simulink model "Xl_ch16_LPF_int_v4"  (Simulink 7.5)
settings: Solver=VariableStepDiscrete  StartTime=0.0  StopTime=0.001  RelTol=1e-3
values from neighbouring files (symbols this model uses):
  a2a = zeros(nFc, length(Hd.sosMatrix(:,5)))    [iirButter_SOS_init_v2.m]    (also in iirButter_SOS_init_v2_8pole.m)
  a3a = zeros(nFc, length(Hd.sosMatrix(:,6)))    [iirButter_SOS_init_v2.m]    (also in iirButter_SOS_init_v2_8pole.m)
  dt = 1/Fsim    (= 2.56e-06)    [iirButter_SOS_init_v2.m]    (also in iirButter_SOS_init_v2_8pole.m)
  Fc_min = 10    [iirButter_SOS_init_v2.m]    (also in iirButter_SOS_init_v2_8pole.m)
  ga = zeros(nFc, length(Hd.ScaleValues))    [iirButter_SOS_init_v2.m]    (also in iirButter_SOS_init_v2_8pole.m = zeros(nFc, length(Hd.ScaleValues(1:end-1))))
  rFc = (Fc_max/Fc_min)^(1/(nFc - 1))    (= 1.70532863139)    [iirButter_SOS_init_v2.m]    (also in iirButter_SOS_init_v2_8pole.m)
  Sra = 2^34|.02  |.027 |.027 |<.038| 1e-6|<2e-6|<2e-6|<2e-6|<2e-6| 8e-6|    [iirButter_SOS_init_v2.m]    (also in iirButter_SOS_init_v2_8pole.m)
  Srm = 2^34|     |     |     |     |     |     |     |     |     |  to |    [iirButter_SOS_init_v2.m]    (also in iirButter_SOS_init_v2_8pole.m)
libraries: xbsIndex_r4 x296, dspsrcs4 x16, simulink x9
(part 2 of 2)

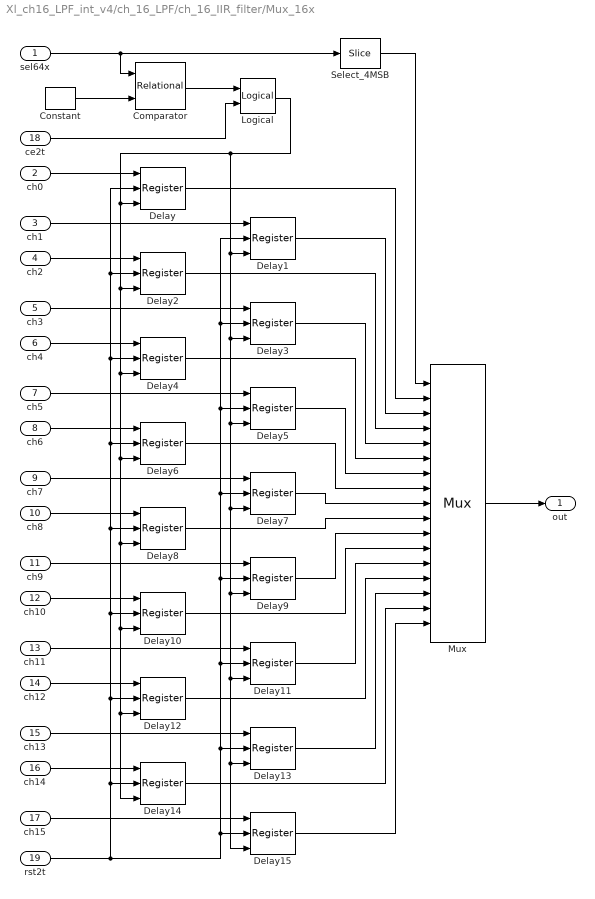
== system Xl_ch16_LPF_int_v4/ch_16_LPF/ch_16_IIR_filter/Mux_16x ==
  sel64x : Inport  OutDataType=fixdt(1, 16)  OutScaling=2^0
  ch0 : Inport  Port=2  OutDataType=fixdt(1, 16)  OutScaling=2^0
  ch1 : Inport  Port=3  OutDataType=fixdt(1, 16)  OutScaling=2^0
  ch2 : Inport  Port=4  OutDataType=fixdt(1, 16)  OutScaling=2^0
  ch3 : Inport  Port=5  OutDataType=fixdt(1, 16)  OutScaling=2^0
  ch4 : Inport  Port=6  OutDataType=fixdt(1, 16)  OutScaling=2^0
  ch5 : Inport  Port=7  OutDataType=fixdt(1, 16)  OutScaling=2^0
  ch6 : Inport  Port=8  OutDataType=fixdt(1, 16)  OutScaling=2^0
  ch7 : Inport  Port=9  OutDataType=fixdt(1, 16)  OutScaling=2^0
  ch8 : Inport  Port=10  OutDataType=fixdt(1, 16)  OutScaling=2^0
  ch9 : Inport  Port=11  OutDataType=fixdt(1, 16)  OutScaling=2^0
  ch10 : Inport  Port=12  OutDataType=fixdt(1, 16)  OutScaling=2^0
  ch11 : Inport  Port=13  OutDataType=fixdt(1, 16)  OutScaling=2^0
  ch12 : Inport  Port=14  OutDataType=fixdt(1, 16)  OutScaling=2^0
  ch13 : Inport  Port=15  OutDataType=fixdt(1, 16)  OutScaling=2^0
  ch14 : Inport  Port=16  OutDataType=fixdt(1, 16)  OutScaling=2^0
  ch15 : Inport  Port=17  OutDataType=fixdt(1, 16)  OutScaling=2^0
  ce2t : Inport  Port=18  OutDataType=fixdt(1, 16)  OutScaling=2^0
  rst2t : Inport  Port=19  OutDataType=fixdt(1, 16)  OutScaling=2^0
  Comparator : xbsIndex_r4/Relational  mode=a=b  en=off  latency=0  dbl_ovrd=off  block_type=relational
      settings: block_version=12.2
  Constant : xbsIndex_r4/Constant  arith_type=Unsigned  const=63  n_bits=6  bin_pt=0  explicit_period=off  period=1  equ=P=C  opselect=C  inp2=PCIN>>17  opr=+  inp1=P  carry=CIN  dbl_ovrd=off  block_type=constant
      settings: block_version=12.2
  Delay{,1..15} (16 alike) : xbsIndex_r4/Register  init=0  rst=on  en=on  dbl_ovrd=off  block_type=register
      settings: block_version=12.2
  Logical : xbsIndex_r4/Logical  logical_function=AND  inputs=2  en=off  latency=0  precision=Full  arith_type=Unsigned  n_bits=16  bin_pt=0  align_bp=on  dbl_ovrd=off  block_type=logical
      settings: block_version=12.2
  Mux : xbsIndex_r4/Mux  inputs=16  en=off  latency=0  precision=Full  arith_type=Unsigned  n_bits=16  bin_pt=14  quantization=Truncate  overflow=Wrap  dbl_ovrd=off  block_type=mux
      settings: block_version=12.2
  Select_4MSB : xbsIndex_r4/Slice  nbits=4  boolean_output=off  mode=Upper Bit Location + Width  bit1=0  base1=MSB of Input  bit0=0  base0=LSB of Input  dbl_ovrd=off  block_type=slice
      settings: block_version=12.2
  out : Outport  OutDataType=fixdt(1, 16)  OutScaling=2^0
  wires:
  Select_4MSB/1 -> Mux/1
  Delay14/1 -> Mux/16
  Delay13/1 -> Mux/15
  Delay12/1 -> Mux/14
  Delay11/1 -> Mux/13
  Delay10/1 -> Mux/12
  Delay9/1 -> Mux/11
  Delay1/1 -> Mux/3
  Delay2/1 -> Mux/4
  Delay3/1 -> Mux/5
  Delay4/1 -> Mux/6
  Delay5/1 -> Mux/7
  Delay6/1 -> Mux/8
  Delay7/1 -> Mux/9
  Delay8/1 -> Mux/10
  Delay/1 -> Mux/2
  Delay15/1 -> Mux/17
  rst2t/1 -> Delay14/2, Delay12/2, Delay10/2, Delay8/2, Delay6/2, Delay4/2, Delay2/2, Delay/2, Delay3/2, Delay1/2, Delay5/2, Delay7/2, Delay9/2, Delay11/2, Delay13/2, Delay15/2
  Logical/1 -> Delay/3, Delay2/3, Delay4/3, Delay6/3, Delay8/3, Delay10/3, Delay12/3, Delay14/3, Delay13/3, Delay15/3, Delay11/3, Delay9/3, Delay7/3, Delay5/3, Delay3/3, Delay1/3
  ce2t/1 -> Logical/2
  Comparator/1 -> Logical/1
  ch15/1 -> Delay15/1
  ch14/1 -> Delay14/1
  ch13/1 -> Delay13/1
  ch12/1 -> Delay12/1
  ch11/1 -> Delay11/1
  ch10/1 -> Delay10/1
  ch9/1 -> Delay9/1
  ch8/1 -> Delay8/1
  ch7/1 -> Delay7/1
  ch6/1 -> Delay6/1
  ch5/1 -> Delay5/1
  ch4/1 -> Delay4/1
  sel64x/1 -> Comparator/1, Select_4MSB/1
  ch3/1 -> Delay3/1
  ch2/1 -> Delay2/1
  ch1/1 -> Delay1/1
  ch0/1 -> Delay/1
  Mux/1 -> out/1
  Constant/1 -> Comparator/2

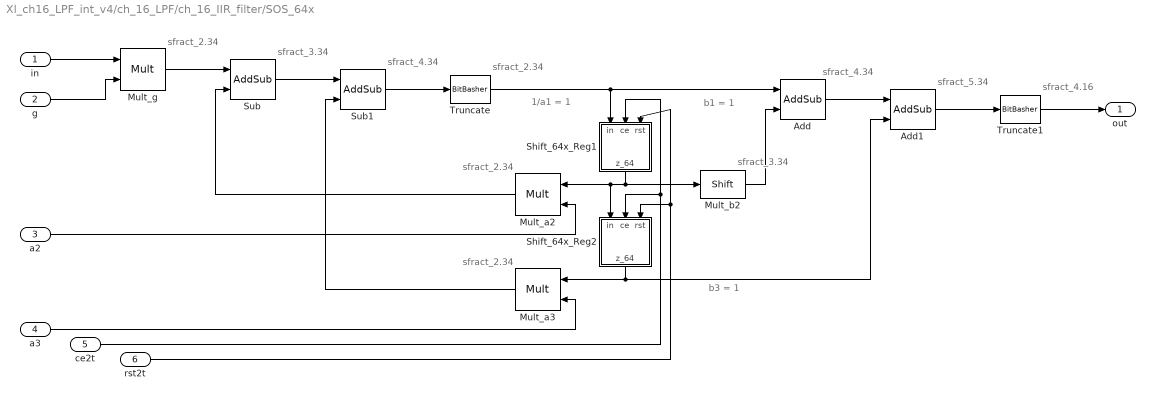
== system Xl_ch16_LPF_int_v4/ch_16_LPF/ch_16_IIR_filter/SOS_64x ==
  note: b1 = 1
  note: b3 = 1
  note: 1/a1 = 1
  note: sfract_3.34
  note: sfract_4.34
  note: sfract_2.34
  note: sfract_3.34
  note: sfract_4.34
  note: sfract_2.34
  note: sfract_2.34
  note: sfract_2.34
  note: sfract_5.34
  note: sfract_4.16
  in : Inport
  g : Inport  Port=2
  a2 : Inport  Port=3
  a3 : Inport  Port=4
  ce2t : Inport  Port=5
  rst2t : Inport  Port=6
  Add : xbsIndex_r4/AddSub  mode=Addition  use_carryin=off  use_carryout=off  en=off  latency=0  precision=Full  arith_type=Unsigned  n_bits=16  bin_pt=14  quantization=Truncate  overflow=Wrap  dbl_ovrd=off  use_behavioral_HDL=off  hw_selection=Fabric  pipelined=off  block_type=addsub
      settings: block_version=12.2
  Add1 : xbsIndex_r4/AddSub  mode=Addition  use_carryin=off  use_carryout=off  en=off  latency=0  precision=Full  arith_type=Unsigned  n_bits=16  bin_pt=14  quantization=Truncate  overflow=Wrap  dbl_ovrd=off  use_behavioral_HDL=off  hw_selection=Fabric  pipelined=off  block_type=addsub
      settings: block_version=12.2
  Mult_a2 : xbsIndex_r4/Mult  precision=User Defined  arith_type="Signed  (2's comp)"  n_bits=36  bin_pt=34  quantization=Truncate  overflow=Wrap  en=off  latency=0  dbl_ovrd=off  use_behavioral_HDL=off  opt=Speed  use_embedded=on  optimum_pipeline=off  pipeline=on  use_rpm=on  placement_style=Triangular  block_type=mult
      settings: block_version=12.2
  Mult_a3 : xbsIndex_r4/Mult  precision=User Defined  arith_type="Signed  (2's comp)"  n_bits=36  bin_pt=34  quantization=Truncate  overflow=Wrap  en=off  latency=0  dbl_ovrd=off  use_behavioral_HDL=off  opt=Speed  use_embedded=on  optimum_pipeline=off  pipeline=on  use_rpm=on  placement_style=Triangular  block_type=mult
      settings: block_version=12.2
  Mult_b2 : xbsIndex_r4/Shift  shift_dir=Left  shift_bits=1  en=off  latency=0  precision=User Defined  arith_type="Signed  (2's comp)"  n_bits=37  bin_pt=34  quantization=Truncate  overflow=Wrap  dbl_ovrd=off  block_type=shift
      settings: block_version=12.2
  Mult_g : xbsIndex_r4/Mult  precision=User Defined  arith_type="Signed  (2's comp)"  n_bits=36  bin_pt=34  quantization=Truncate  overflow=Wrap  en=off  latency=0  dbl_ovrd=off  use_behavioral_HDL=off  opt=Speed  use_embedded=on  optimum_pipeline=off  pipeline=on  use_rpm=on  placement_style=Triangular  block_type=mult
      settings: block_version=12.2
  Shift_64x_Reg1 : Subsystem
  Shift_64x_Reg2 : Subsystem
  Sub : xbsIndex_r4/AddSub  mode=Subtraction  use_carryin=off  use_carryout=off  en=off  latency=0  precision=Full  arith_type=Unsigned  n_bits=16  bin_pt=14  quantization=Truncate  overflow=Wrap  dbl_ovrd=off  use_behavioral_HDL=off  hw_selection=Fabric  pipelined=off  block_type=addsub
      settings: block_version=12.2
  Sub1 : xbsIndex_r4/AddSub  mode=Subtraction  use_carryin=off  use_carryout=off  en=off  latency=0  precision=Full  arith_type=Unsigned  n_bits=16  bin_pt=14  quantization=Truncate  overflow=Wrap  dbl_ovrd=off  use_behavioral_HDL=off  hw_selection=Fabric  pipelined=off  block_type=addsub
      settings: block_version=12.2
  Truncate : xbsIndex_r4/BitBasher  bitexpr=|  display_expr=off  sr_1=1  arith_type1="Signed  (2's comp)"  bin_pt1=34  sr_2=2  arith_type2=Unsigned  bin_pt2=0  sr_3=3  arith_type3=Unsigned  bin_pt3=0  sr_4=4  arith_type4=Unsigned  bin_pt4=0  dbl_ovrd=off  block_type=bitbasher
      | <!DOCTYPE HTML PUBLIC "-//W3C//DTD HTML 4.0//EN" "http://www.w3.org/TR/REC-html40/strict.dtd">
      | <html><head><meta name="qrichtext" content="1" /><style type="text/css">
      | p, li { white-space: pre-wrap; }
      | </style></head><body style=" font-family:'MS Shell Dlg 2'; font-size:8.25pt; font-weight:400; font-style:normal;">
      | <p style=" margin-top:12px; margin-bottom:12px; margin-left:0px; margin-right:0px; -qt-block-indent:0; text-indent:0px; font-family:'MS Shell Dlg'; font-size:8pt;">a={b[35:0]}</p></body></html>
      settings: block_version=12.2
  Truncate1 : xbsIndex_r4/BitBasher  bitexpr=|  display_expr=off  sr_1=1  arith_type1="Signed  (2's comp)"  bin_pt1=16  sr_2=2  arith_type2=Unsigned  bin_pt2=0  sr_3=3  arith_type3=Unsigned  bin_pt3=0  sr_4=4  arith_type4=Unsigned  bin_pt4=0  dbl_ovrd=off  block_type=bitbasher
      | <!DOCTYPE HTML PUBLIC "-//W3C//DTD HTML 4.0//EN" "http://www.w3.org/TR/REC-html40/strict.dtd">
      | <html><head><meta name="qrichtext" content="1" /><style type="text/css">
      | p, li { white-space: pre-wrap; }
      | </style></head><body style=" font-family:'MS Shell Dlg 2'; font-size:8.25pt; font-weight:400; font-style:normal;">
      | <p style=" margin-top:12px; margin-bottom:12px; margin-left:0px; margin-right:0px; -qt-block-indent:0; text-indent:0px; font-family:'MS Shell Dlg'; font-size:8pt;">a={b[37:18]}</p></body></html>
      settings: block_version=12.2
  out : Outport
  wires:
  a3/1 -> Mult_a3/2
  a2/1 -> Mult_a2/2
  g/1 -> Mult_g/2
  Shift_64x_Reg1/1(z_64) -> Mult_a2/1, Shift_64x_Reg2/1(in), Mult_b2/1
  Mult_b2/1 -> Add/2
  Shift_64x_Reg2/1(z_64) -> Mult_a3/1, Add1/2
  Sub1/1 -> Truncate/1
  Mult_a2/1 -> Sub/2
  Mult_a3/1 -> Sub1/2
  Mult_g/1 -> Sub/1
  in/1 -> Mult_g/1
  Add1/1 -> Truncate1/1
  Truncate/1 -> Add/1, Shift_64x_Reg1/1(in)
  Truncate1/1 -> out/1
  Add/1 -> Add1/1
  Sub/1 -> Sub1/1
  ce2t/1 -> Shift_64x_Reg1/2(ce), Shift_64x_Reg2/2(ce)
  rst2t/1 -> Shift_64x_Reg1/3(rst), Shift_64x_Reg2/3(rst)

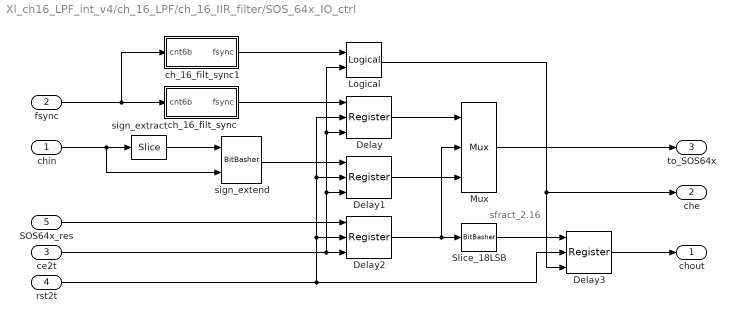
== system Xl_ch16_LPF_int_v4/ch_16_LPF/ch_16_IIR_filter/SOS_64x_IO_ctrl ==
  note: sfract_2.16
  chin : Inport  OutDataType=fixdt(1, 16)  OutScaling=2^0
  fsync : Inport  Port=2  OutDataType=fixdt(1, 16)  OutScaling=2^0
  ce2t : Inport  Port=3  OutDataType=fixdt(1, 16)  OutScaling=2^0
  rst2t : Inport  Port=4  OutDataType=fixdt(1, 16)  OutScaling=2^0
  SOS64x_res : Inport  Port=5  OutDataType=fixdt(1, 16)  OutScaling=2^0
  Delay{,1..3} (4 alike) : xbsIndex_r4/Register  init=0  rst=on  en=on  dbl_ovrd=off  block_type=register
      settings: block_version=12.2
  Logical : xbsIndex_r4/Logical  logical_function=AND  inputs=2  en=off  latency=0  precision=Full  arith_type=Unsigned  n_bits=16  bin_pt=0  align_bp=on  dbl_ovrd=off  block_type=logical
      settings: block_version=12.2
  Mux : xbsIndex_r4/Mux  inputs=2  en=off  latency=0  precision=Full  arith_type=Unsigned  n_bits=16  bin_pt=14  quantization=Truncate  overflow=Wrap  dbl_ovrd=off  block_type=mux
      settings: block_version=12.2
  Slice_18LSB : xbsIndex_r4/BitBasher  bitexpr=|  display_expr=off  sr_1=1  arith_type1="Signed  (2's comp)"  bin_pt1=16  sr_2=2  arith_type2=Unsigned  bin_pt2=0  sr_3=3  arith_type3=Unsigned  bin_pt3=0  sr_4=4  arith_type4=Unsigned  bin_pt4=0  dbl_ovrd=off  block_type=bitbasher
      | <!DOCTYPE HTML PUBLIC "-//W3C//DTD HTML 4.0//EN" "http://www.w3.org/TR/REC-html40/strict.dtd">
      | <html><head><meta name="qrichtext" content="1" /><style type="text/css">
      | p, li { white-space: pre-wrap; }
      | </style></head><body style=" font-family:'MS Shell Dlg 2'; font-size:8.25pt; font-weight:400; font-style:normal;">
      | <p style=" margin-top:12px; margin-bottom:12px; margin-left:0px; margin-right:0px; -qt-block-indent:0; text-indent:0px; font-family:'MS Shell Dlg'; font-size:8pt;">a={b[17:0]}</p></body></html>
      settings: block_version=12.2
  ch_16_filt_sync : Subsystem
  ch_16_filt_sync1 : Subsystem
  sign_extend : xbsIndex_r4/BitBasher  bitexpr=|  display_expr=off  sr_1=1  arith_type1="Signed  (2's comp)"  bin_pt1=16  sr_2=2  arith_type2=Unsigned  bin_pt2=0  sr_3=3  arith_type3=Unsigned  bin_pt3=0  sr_4=4  arith_type4=Unsigned  bin_pt4=0  dbl_ovrd=off  block_type=bitbasher
      | <!DOCTYPE HTML PUBLIC "-//W3C//DTD HTML 4.0//EN" "http://www.w3.org/TR/REC-html40/strict.dtd">
      | <html><head><meta name="qrichtext" content="1" /><style type="text/css">
      | p, li { white-space: pre-wrap; }
      | </style></head><body style=" font-family:'MS Shell Dlg 2'; font-size:8.25pt; font-weight:400; font-style:normal;">
      | <p style=" margin-top:12px; margin-bottom:12px; margin-left:0px; margin-right:0px; -qt-block-indent:0; text-indent:0px; font-family:'MS Shell Dlg'; font-size:8pt;">a={2{b},c}</p></body></html>
      settings: block_version=12.2
  sign_extract : xbsIndex_r4/Slice  nbits=1  boolean_output=on  mode=Upper Bit Location + Width  bit1=0  base1=MSB of Input  bit0=0  base0=LSB of Input  dbl_ovrd=off  block_type=slice
      settings: block_version=12.2
  chout : Outport  OutDataType=fixdt(1, 16)  OutScaling=2^0
  che : Outport  Port=2  OutDataType=fixdt(1, 16)  OutScaling=2^0
  to_SOS64x : Outport  Port=3  OutDataType=fixdt(1, 16)  OutScaling=2^0
  wires:
  fsync/1 -> ch_16_filt_sync/1(cnt6b), ch_16_filt_sync1/1(cnt6b)
  Delay/1 -> Mux/1
  Delay1/1 -> Mux/3
  chin/1 -> sign_extract/1, sign_extend/2
  Delay2/1 -> Mux/2, Slice_18LSB/1
  SOS64x_res/1 -> Delay2/1
  Mux/1 -> to_SOS64x/1
  Logical/1 -> Delay3/3, che/1
  ce2t/1 -> Delay2/3, Delay/3, Logical/2, Delay1/3
  rst2t/1 -> Delay/2, Delay1/2, Delay2/2, Delay3/2
  sign_extend/1 -> Delay1/1
  sign_extract/1 -> sign_extend/1
  Slice_18LSB/1 -> Delay3/1
  ch_16_filt_sync/1(fsync) -> Delay/1
  ch_16_filt_sync1/1(fsync) -> Logical/1
  Delay3/1 -> chout/1

== system Xl_ch16_LPF_int_v4/ch_16_LPF/ch_16_IIR_filter/Subsystem ==
  In1 : Inport
  Time Division Demultiplexer : xbsIndex_r4/Time Division Demultiplexer  frame_pattern=[1 0]  impl_style=Multiple Channel  vin=off  dbl_ovrd=off  explicit_period=off  period=1  block_type=tdd
      settings: infoedit=Samples presented at the input are selected and down-sampled according to the frame sampling pattern specified. The sampled input is presented either as a single or multiple channel at the output.  block_version=12.2
  Time Division Demultiplexer1 : xbsIndex_r4/Time Division Demultiplexer  frame_pattern=[0 0 0 1 1 0 0 0 zeros(1,24)]  impl_style=Multiple Channel  vin=off  dbl_ovrd=off  explicit_period=off  period=1  block_type=tdd
      settings: infoedit=Samples presented at the input are selected and down-sampled according to the frame sampling pattern specified. The sampled input is presented either as a single or multiple channel at the output.  block_version=12.2
  Time Division Demultiplexer2 : xbsIndex_r4/Time Division Demultiplexer  frame_pattern=[1 1]  impl_style=Multiple Channel  vin=off  dbl_ovrd=off  explicit_period=off  period=1  block_type=tdd
      settings: infoedit=Samples presented at the input are selected and down-sampled according to the frame sampling pattern specified. The sampled input is presented either as a single or multiple channel at the output.  block_version=12.2
  Time Division Demultiplexer3 : xbsIndex_r4/Time Division Demultiplexer  frame_pattern=[0 0 0 1 1 0 0 0 zeros(1,24)]  impl_style=Multiple Channel  vin=off  dbl_ovrd=off  explicit_period=off  period=1  block_type=tdd
      settings: infoedit=Samples presented at the input are selected and down-sampled according to the frame sampling pattern specified. The sampled input is presented either as a single or multiple channel at the output.  block_version=12.2
  Out1 : Outport
  Out2 : Outport  Port=2
  Out3 : Outport  Port=3
  Out4 : Outport  Port=4
  wires:
  Time Division Demultiplexer/1 -> Time Division Demultiplexer2/1
  Time Division Demultiplexer2/1 -> Time Division Demultiplexer1/1
  Time Division Demultiplexer2/2 -> Time Division Demultiplexer3/1
  Time Division Demultiplexer1/1 -> Out1/1
  In1/1 -> Time Division Demultiplexer/1
  Time Division Demultiplexer1/2 -> Out2/1
  Time Division Demultiplexer3/1 -> Out3/1
  Time Division Demultiplexer3/2 -> Out4/1

== system Xl_ch16_LPF_int_v4/ch_16_LPF/ch_16_IIR_filter/Subsystem1 ==
  In1 : Inport
  Time Division Demultiplexer : xbsIndex_r4/Time Division Demultiplexer  frame_pattern=[1 0]  impl_style=Multiple Channel  vin=off  dbl_ovrd=off  explicit_period=off  period=1  block_type=tdd
      settings: infoedit=Samples presented at the input are selected and down-sampled according to the frame sampling pattern specified. The sampled input is presented either as a single or multiple channel at the output.  block_version=12.2
  Time Division Demultiplexer1 : xbsIndex_r4/Time Division Demultiplexer  frame_pattern=[0 0 0 1 1 0 0 0 zeros(1,24)]  impl_style=Multiple Channel  vin=off  dbl_ovrd=off  explicit_period=off  period=1  block_type=tdd
      settings: infoedit=Samples presented at the input are selected and down-sampled according to the frame sampling pattern specified. The sampled input is presented either as a single or multiple channel at the output.  block_version=12.2
  Time Division Demultiplexer2 : xbsIndex_r4/Time Division Demultiplexer  frame_pattern=[1 1]  impl_style=Multiple Channel  vin=off  dbl_ovrd=off  explicit_period=off  period=1  block_type=tdd
      settings: infoedit=Samples presented at the input are selected and down-sampled according to the frame sampling pattern specified. The sampled input is presented either as a single or multiple channel at the output.  block_version=12.2
  Time Division Demultiplexer3 : xbsIndex_r4/Time Division Demultiplexer  frame_pattern=[0 0 0 1 1 0 0 0 zeros(1,24)]  impl_style=Multiple Channel  vin=off  dbl_ovrd=off  explicit_period=off  period=1  block_type=tdd
      settings: infoedit=Samples presented at the input are selected and down-sampled according to the frame sampling pattern specified. The sampled input is presented either as a single or multiple channel at the output.  block_version=12.2
  Out1 : Outport
  Out2 : Outport  Port=2
  Out3 : Outport  Port=3
  Out4 : Outport  Port=4
  wires:
  Time Division Demultiplexer/1 -> Time Division Demultiplexer2/1
  Time Division Demultiplexer2/1 -> Time Division Demultiplexer1/1
  Time Division Demultiplexer2/2 -> Time Division Demultiplexer3/1
  Time Division Demultiplexer1/1 -> Out1/1
  In1/1 -> Time Division Demultiplexer/1
  Time Division Demultiplexer1/2 -> Out2/1
  Time Division Demultiplexer3/1 -> Out3/1
  Time Division Demultiplexer3/2 -> Out4/1

== system Xl_ch16_LPF_int_v4/ch_16_LPF/ch_16_IIR_filter/Subsystem2 ==
  In1 : Inport
  Time Division Demultiplexer : xbsIndex_r4/Time Division Demultiplexer  frame_pattern=[1 0]  impl_style=Multiple Channel  vin=off  dbl_ovrd=off  explicit_period=off  period=1  block_type=tdd
      settings: infoedit=Samples presented at the input are selected and down-sampled according to the frame sampling pattern specified. The sampled input is presented either as a single or multiple channel at the output.  block_version=12.2
  Time Division Demultiplexer1 : xbsIndex_r4/Time Division Demultiplexer  frame_pattern=[0 0 0 1 1 1 0 0 zeros(1,24)]  impl_style=Multiple Channel  vin=off  dbl_ovrd=off  explicit_period=off  period=1  block_type=tdd
      settings: infoedit=Samples presented at the input are selected and down-sampled according to the frame sampling pattern specified. The sampled input is presented either as a single or multiple channel at the output.  block_version=12.2
  Time Division Demultiplexer2 : xbsIndex_r4/Time Division Demultiplexer  frame_pattern=[1 1]  impl_style=Multiple Channel  vin=off  dbl_ovrd=off  explicit_period=off  period=1  block_type=tdd
      settings: infoedit=Samples presented at the input are selected and down-sampled according to the frame sampling pattern specified. The sampled input is presented either as a single or multiple channel at the output.  block_version=12.2
  Time Division Demultiplexer3 : xbsIndex_r4/Time Division Demultiplexer  frame_pattern=[0 0 0 1 1 1 0 0 zeros(1,24)]  impl_style=Multiple Channel  vin=off  dbl_ovrd=off  explicit_period=off  period=1  block_type=tdd
      settings: infoedit=Samples presented at the input are selected and down-sampled according to the frame sampling pattern specified. The sampled input is presented either as a single or multiple channel at the output.  block_version=12.2
  Out1 : Outport
  Out2 : Outport  Port=2
  Out3 : Outport  Port=3
  Out4 : Outport  Port=4
  Out5 : Outport  Port=5
  Out6 : Outport  Port=6
  wires:
  Time Division Demultiplexer/1 -> Time Division Demultiplexer2/1
  Time Division Demultiplexer2/1 -> Time Division Demultiplexer1/1
  Time Division Demultiplexer2/2 -> Time Division Demultiplexer3/1
  Time Division Demultiplexer1/1 -> Out1/1
  In1/1 -> Time Division Demultiplexer/1
  Time Division Demultiplexer1/2 -> Out2/1
  Time Division Demultiplexer3/1 -> Out3/1
  Time Division Demultiplexer3/2 -> Out4/1
  Time Division Demultiplexer1/3 -> Out5/1
  Time Division Demultiplexer3/3 -> Out6/1

== system Xl_ch16_LPF_int_v4/ch_16_LPF/ch_16_IIR_filter/ch_16_filt_sync1 ==
  cnt6b : Inport  OutDataType=fixdt(1, 16)  OutScaling=2^0
  ce2t : Inport  Port=2  OutDataType=fixdt(1, 16)  OutScaling=2^0
  AeqB : xbsIndex_r4/Relational  mode=a=b  en=off  latency=0  dbl_ovrd=off  block_type=relational
      settings: block_version=12.2
  Constant : xbsIndex_r4/Constant  arith_type=Unsigned  const=2  n_bits=2  bin_pt=0  explicit_period=off  period=1  equ=P=C  opselect=C  inp2=PCIN>>17  opr=+  inp1=P  carry=CIN  dbl_ovrd=off  block_type=constant
      settings: block_version=12.2
  Logical : xbsIndex_r4/Logical  logical_function=AND  inputs=2  en=off  latency=0  precision=Full  arith_type=Unsigned  n_bits=16  bin_pt=0  align_bp=on  dbl_ovrd=off  block_type=logical
      settings: block_version=12.2
  Slice_2LSB : xbsIndex_r4/Slice  nbits=2  boolean_output=off  mode=Lower Bit Location + Width  bit1=0  base1=MSB of Input  bit0=0  base0=LSB of Input  dbl_ovrd=off  block_type=slice
      settings: block_version=12.2
  fsync : Outport  OutDataType=fixdt(1, 16)  OutScaling=2^0
  che : Outport  Port=2  OutDataType=fixdt(1, 16)  OutScaling=2^0
  wires:
  cnt6b/1 -> Slice_2LSB/1
  Slice_2LSB/1 -> AeqB/1
  AeqB/1 -> fsync/1, Logical/1
  Constant/1 -> AeqB/2
  ce2t/1 -> Logical/2
  Logical/1 -> che/1

== system Xl_ch16_LPF_int_v4/ch_16_LPF/ch_16_IIR_filter/Demux_16x/Subsystem1 ==
  In1 : Inport
  Time Division Demultiplexer : xbsIndex_r4/Time Division Demultiplexer  frame_pattern=[1 0]  impl_style=Multiple Channel  vin=off  dbl_ovrd=off  explicit_period=off  period=1  block_type=tdd
      settings: infoedit=Samples presented at the input are selected and down-sampled according to the frame sampling pattern specified. The sampled input is presented either as a single or multiple channel at the output.  block_version=12.2
  Time Division Demultiplexer1 : xbsIndex_r4/Time Division Demultiplexer  frame_pattern=[0 0 0 1 1 1 0 0 zeros(1,24)]  impl_style=Multiple Channel  vin=off  dbl_ovrd=off  explicit_period=off  period=1  block_type=tdd
      settings: infoedit=Samples presented at the input are selected and down-sampled according to the frame sampling pattern specified. The sampled input is presented either as a single or multiple channel at the output.  block_version=12.2
  Time Division Demultiplexer2 : xbsIndex_r4/Time Division Demultiplexer  frame_pattern=[1 1]  impl_style=Multiple Channel  vin=off  dbl_ovrd=off  explicit_period=off  period=1  block_type=tdd
      settings: infoedit=Samples presented at the input are selected and down-sampled according to the frame sampling pattern specified. The sampled input is presented either as a single or multiple channel at the output.  block_version=12.2
  Time Division Demultiplexer3 : xbsIndex_r4/Time Division Demultiplexer  frame_pattern=[0 0 0 1 1 1 0 0 zeros(1,24)]  impl_style=Multiple Channel  vin=off  dbl_ovrd=off  explicit_period=off  period=1  block_type=tdd
      settings: infoedit=Samples presented at the input are selected and down-sampled according to the frame sampling pattern specified. The sampled input is presented either as a single or multiple channel at the output.  block_version=12.2
  Out1 : Outport
  Out2 : Outport  Port=2
  Out3 : Outport  Port=3
  Out4 : Outport  Port=4
  Out5 : Outport  Port=5
  Out6 : Outport  Port=6
  wires:
  Time Division Demultiplexer/1 -> Time Division Demultiplexer2/1
  Time Division Demultiplexer2/1 -> Time Division Demultiplexer1/1
  Time Division Demultiplexer2/2 -> Time Division Demultiplexer3/1
  Time Division Demultiplexer1/1 -> Out1/1
  In1/1 -> Time Division Demultiplexer/1
  Time Division Demultiplexer1/2 -> Out2/1
  Time Division Demultiplexer3/1 -> Out3/1
  Time Division Demultiplexer3/2 -> Out4/1
  Time Division Demultiplexer1/3 -> Out5/1
  Time Division Demultiplexer3/3 -> Out6/1

== system Xl_ch16_LPF_int_v4/ch_16_LPF/ch_16_IIR_filter/Demux_16x/Subsystem3 ==
  In1 : Inport
  Time Division Demultiplexer : xbsIndex_r4/Time Division Demultiplexer  frame_pattern=[1 0]  impl_style=Multiple Channel  vin=off  dbl_ovrd=off  explicit_period=off  period=1  block_type=tdd
      settings: infoedit=Samples presented at the input are selected and down-sampled according to the frame sampling pattern specified. The sampled input is presented either as a single or multiple channel at the output.  block_version=12.2
  Time Division Demultiplexer1 : xbsIndex_r4/Time Division Demultiplexer  frame_pattern=[0 0 0 1 1 1 0 0 zeros(1,24)]  impl_style=Multiple Channel  vin=off  dbl_ovrd=off  explicit_period=off  period=1  block_type=tdd
      settings: infoedit=Samples presented at the input are selected and down-sampled according to the frame sampling pattern specified. The sampled input is presented either as a single or multiple channel at the output.  block_version=12.2
  Time Division Demultiplexer2 : xbsIndex_r4/Time Division Demultiplexer  frame_pattern=[1 1]  impl_style=Multiple Channel  vin=off  dbl_ovrd=off  explicit_period=off  period=1  block_type=tdd
      settings: infoedit=Samples presented at the input are selected and down-sampled according to the frame sampling pattern specified. The sampled input is presented either as a single or multiple channel at the output.  block_version=12.2
  Time Division Demultiplexer3 : xbsIndex_r4/Time Division Demultiplexer  frame_pattern=[0 0 0 1 1 1 0 0 zeros(1,24)]  impl_style=Multiple Channel  vin=off  dbl_ovrd=off  explicit_period=off  period=1  block_type=tdd
      settings: infoedit=Samples presented at the input are selected and down-sampled according to the frame sampling pattern specified. The sampled input is presented either as a single or multiple channel at the output.  block_version=12.2
  Out1 : Outport
  Out2 : Outport  Port=2
  Out3 : Outport  Port=3
  Out4 : Outport  Port=4
  Out5 : Outport  Port=5
  Out6 : Outport  Port=6
  wires:
  Time Division Demultiplexer/1 -> Time Division Demultiplexer2/1
  Time Division Demultiplexer2/1 -> Time Division Demultiplexer1/1
  Time Division Demultiplexer2/2 -> Time Division Demultiplexer3/1
  Time Division Demultiplexer1/1 -> Out1/1
  In1/1 -> Time Division Demultiplexer/1
  Time Division Demultiplexer1/2 -> Out2/1
  Time Division Demultiplexer3/1 -> Out3/1
  Time Division Demultiplexer3/2 -> Out4/1
  Time Division Demultiplexer1/3 -> Out5/1
  Time Division Demultiplexer3/3 -> Out6/1

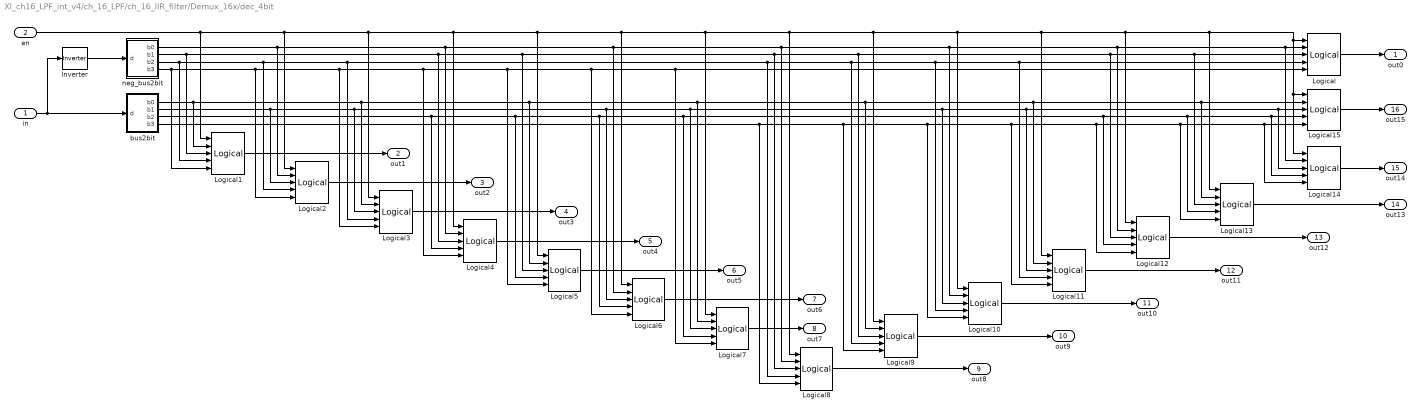
== system Xl_ch16_LPF_int_v4/ch_16_LPF/ch_16_IIR_filter/Demux_16x/dec_4bit ==
  in : Inport  OutDataType=fixdt(1, 16)  OutScaling=2^0
  en : Inport  Port=2  OutDataType=fixdt(1, 16)  OutScaling=2^0
  Inverter : xbsIndex_r4/Inverter  en=off  latency=0  dbl_ovrd=off  block_type=inv
      settings: block_version=12.2
  Logical{,1..15} (16 alike) : xbsIndex_r4/Logical  logical_function=AND  inputs=5  en=off  latency=0  precision=Full  arith_type=Unsigned  n_bits=16  bin_pt=0  align_bp=on  dbl_ovrd=off  block_type=logical
      settings: block_version=12.2
  bus2bit : Subsystem
  neg_bus2bit : Subsystem
  out0 : Outport  OutDataType=fixdt(1, 16)  OutScaling=2^0
  out1 : Outport  Port=2  OutDataType=fixdt(1, 16)  OutScaling=2^0
  out2 : Outport  Port=3  OutDataType=fixdt(1, 16)  OutScaling=2^0
  out3 : Outport  Port=4  OutDataType=fixdt(1, 16)  OutScaling=2^0
  out4 : Outport  Port=5  OutDataType=fixdt(1, 16)  OutScaling=2^0
  out5 : Outport  Port=6  OutDataType=fixdt(1, 16)  OutScaling=2^0
  out6 : Outport  Port=7  OutDataType=fixdt(1, 16)  OutScaling=2^0
  out7 : Outport  Port=8  OutDataType=fixdt(1, 16)  OutScaling=2^0
  out8 : Outport  Port=9  OutDataType=fixdt(1, 16)  OutScaling=2^0
  out9 : Outport  Port=10  OutDataType=fixdt(1, 16)  OutScaling=2^0
  out10 : Outport  Port=11  OutDataType=fixdt(1, 16)  OutScaling=2^0
  out11 : Outport  Port=12  OutDataType=fixdt(1, 16)  OutScaling=2^0
  out12 : Outport  Port=13  OutDataType=fixdt(1, 16)  OutScaling=2^0
  out13 : Outport  Port=14  OutDataType=fixdt(1, 16)  OutScaling=2^0
  out14 : Outport  Port=15  OutDataType=fixdt(1, 16)  OutScaling=2^0
  out15 : Outport  Port=16  OutDataType=fixdt(1, 16)  OutScaling=2^0
  wires:
  Logical14/1 -> out14/1
  Logical13/1 -> out13/1
  Logical12/1 -> out12/1
  Logical11/1 -> out11/1
  Logical10/1 -> out10/1
  Logical9/1 -> out9/1
  Logical8/1 -> out8/1
  Logical7/1 -> out7/1
  Logical6/1 -> out6/1
  Logical5/1 -> out5/1
  Logical4/1 -> out4/1
  Logical3/1 -> out3/1
  Logical2/1 -> out2/1
  Logical1/1 -> out1/1
  en/1 -> Logical15/1, Logical14/1, Logical/1, Logical13/1, Logical12/1, Logical11/1, Logical10/1, Logical9/1, Logical8/1, Logical7/1, Logical6/1, Logical5/1, Logical4/1, Logical3/1, Logical2/1, Logical1/1
  Logical15/1 -> out15/1
  bus2bit/4(b3) -> Logical14/5, Logical15/5, Logical13/5, Logical12/5, Logical11/5, Logical10/5, Logical9/5, Logical8/5
  bus2bit/3(b2) -> Logical14/4, Logical15/4, Logical13/4, Logical12/4, Logical7/4, Logical6/4, Logical5/4, Logical4/4
  bus2bit/2(b1) -> Logical14/3, Logical15/3, Logical11/3, Logical10/3, Logical7/3, Logical6/3, Logical3/3, Logical2/3
  bus2bit/1(b0) -> Logical13/2, Logical15/2, Logical11/2, Logical9/2, Logical7/2, Logical5/2, Logical3/2, Logical1/2
  Logical/1 -> out0/1
  neg_bus2bit/4(b3) -> Logical/5, Logical7/5, Logical6/5, Logical5/5, Logical4/5, Logical3/5, Logical2/5, Logical1/5
  neg_bus2bit/3(b2) -> Logical11/4, Logical/4, Logical10/4, Logical9/4, Logical8/4, Logical3/4, Logical2/4, Logical1/4
  neg_bus2bit/2(b1) -> Logical13/3, Logical/3, Logical12/3, Logical9/3, Logical8/3, Logical5/3, Logical4/3, Logical1/3
  neg_bus2bit/1(b0) -> Logical14/2, Logical/2, Logical12/2, Logical10/2, Logical8/2, Logical6/2, Logical4/2, Logical2/2
  Inverter/1 -> neg_bus2bit/1(d)
  in/1 -> Inverter/1, bus2bit/1(d)

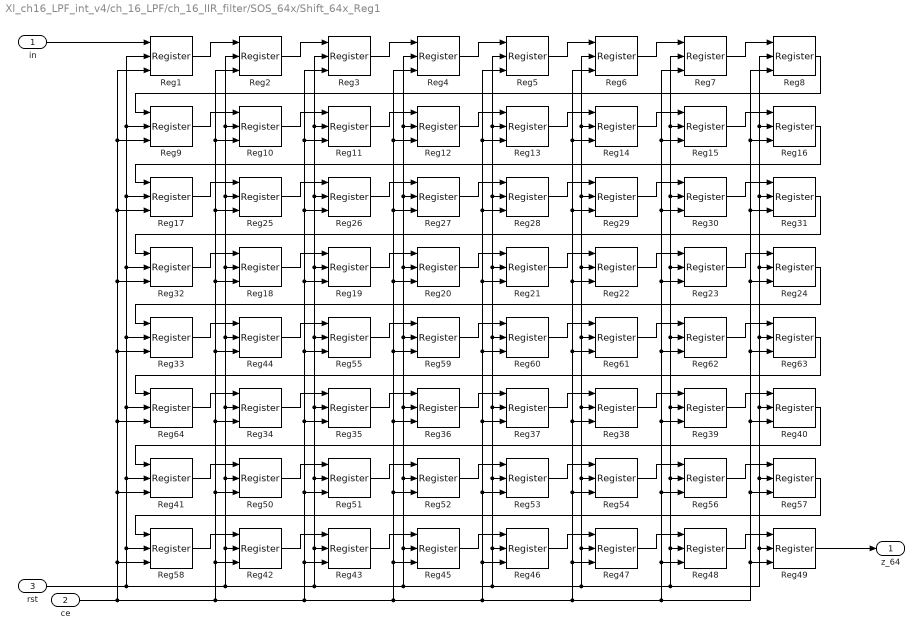
== system Xl_ch16_LPF_int_v4/ch_16_LPF/ch_16_IIR_filter/SOS_64x/Shift_64x_Reg1 ==
  in : Inport  OutDataType=fixdt(1, 16)  OutScaling=2^0
  ce : Inport  Port=2  OutDataType=fixdt(1, 16)  OutScaling=2^0
  rst : Inport  Port=3  OutDataType=fixdt(1, 16)  OutScaling=2^0
  Reg{1..64} (64 alike) : xbsIndex_r4/Register  init=0  rst=on  en=on  dbl_ovrd=off  block_type=register
      settings: block_version=12.2
  z_64 : Outport  OutDataType=fixdt(1, 16)  OutScaling=2^0
  wires:
  Reg7/1 -> Reg8/1
  Reg6/1 -> Reg7/1
  Reg5/1 -> Reg6/1
  Reg4/1 -> Reg5/1
  Reg3/1 -> Reg4/1
  Reg2/1 -> Reg3/1
  Reg1/1 -> Reg2/1
  in/1 -> Reg1/1
  Reg15/1 -> Reg16/1
  Reg14/1 -> Reg15/1
  Reg13/1 -> Reg14/1
  Reg12/1 -> Reg13/1
  Reg11/1 -> Reg12/1
  Reg10/1 -> Reg11/1
  Reg9/1 -> Reg10/1
  Reg8/1 -> Reg9/1
  Reg30/1 -> Reg31/1
  Reg29/1 -> Reg30/1
  Reg28/1 -> Reg29/1
  Reg27/1 -> Reg28/1
  Reg26/1 -> Reg27/1
  Reg25/1 -> Reg26/1
  Reg17/1 -> Reg25/1
  Reg23/1 -> Reg24/1
  Reg22/1 -> Reg23/1
  Reg21/1 -> Reg22/1
  Reg20/1 -> Reg21/1
  Reg19/1 -> Reg20/1
  Reg18/1 -> Reg19/1
  Reg32/1 -> Reg18/1
  Reg31/1 -> Reg32/1
  Reg16/1 -> Reg17/1
  Reg62/1 -> Reg63/1
  Reg61/1 -> Reg62/1
  Reg60/1 -> Reg61/1
  Reg59/1 -> Reg60/1
  Reg55/1 -> Reg59/1
  Reg44/1 -> Reg55/1
  Reg33/1 -> Reg44/1
  Reg39/1 -> Reg40/1
  Reg38/1 -> Reg39/1
  Reg37/1 -> Reg38/1
  Reg36/1 -> Reg37/1
  Reg35/1 -> Reg36/1
  Reg34/1 -> Reg35/1
  Reg64/1 -> Reg34/1
  Reg63/1 -> Reg64/1
  Reg56/1 -> Reg57/1
  Reg54/1 -> Reg56/1
  Reg53/1 -> Reg54/1
  Reg52/1 -> Reg53/1
  Reg51/1 -> Reg52/1
  Reg50/1 -> Reg51/1
  Reg41/1 -> Reg50/1
  Reg48/1 -> Reg49/1
  Reg47/1 -> Reg48/1
  Reg46/1 -> Reg47/1
  Reg45/1 -> Reg46/1
  Reg43/1 -> Reg45/1
  Reg42/1 -> Reg43/1
  Reg58/1 -> Reg42/1
  Reg57/1 -> Reg58/1
  Reg40/1 -> Reg41/1
  Reg24/1 -> Reg33/1
  Reg49/1 -> z_64/1
  rst/1 -> Reg8/2, Reg16/2, Reg31/2, Reg24/2, Reg63/2, Reg40/2, Reg57/2, Reg49/2, Reg7/2, Reg15/2, Reg30/2, Reg23/2, Reg62/2, Reg39/2, Reg56/2, Reg48/2, Reg6/2, Reg14/2, Reg29/2, Reg22/2, Reg61/2, Reg38/2, Reg54/2, Reg47/2, Reg5/2, Reg13/2, Reg28/2, Reg21/2, Reg60/2, Reg37/2, Reg53/2, Reg46/2, Reg4/2, Reg12/2, Reg27/2, Reg20/2, Reg59/2, Reg36/2, Reg52/2, Reg45/2, Reg43/2, Reg51/2, Reg35/2, Reg55/2, Reg19/2, Reg26/2, Reg3/2, Reg11/2, Reg2/2, Reg10/2, Reg25/2, Reg18/2, Reg44/2, Reg34/2, Reg50/2, Reg42/2, Reg1/2, Reg9/2, Reg17/2, Reg32/2, Reg33/2, Reg64/2, Reg41/2, Reg58/2
  ce/1 -> Reg8/3, Reg16/3, Reg31/3, Reg24/3, Reg63/3, Reg40/3, Reg57/3, Reg49/3, Reg7/3, Reg15/3, Reg30/3, Reg23/3, Reg62/3, Reg39/3, Reg56/3, Reg48/3, Reg6/3, Reg14/3, Reg29/3, Reg22/3, Reg61/3, Reg38/3, Reg54/3, Reg47/3, Reg5/3, Reg13/3, Reg28/3, Reg21/3, Reg60/3, Reg37/3, Reg53/3, Reg46/3, Reg4/3, Reg12/3, Reg27/3, Reg20/3, Reg59/3, Reg36/3, Reg52/3, Reg45/3, Reg3/3, Reg11/3, Reg26/3, Reg19/3, Reg55/3, Reg35/3, Reg51/3, Reg43/3, Reg2/3, Reg10/3, Reg25/3, Reg18/3, Reg44/3, Reg34/3, Reg50/3, Reg42/3, Reg1/3, Reg9/3, Reg17/3, Reg32/3, Reg33/3, Reg64/3, Reg41/3, Reg58/3

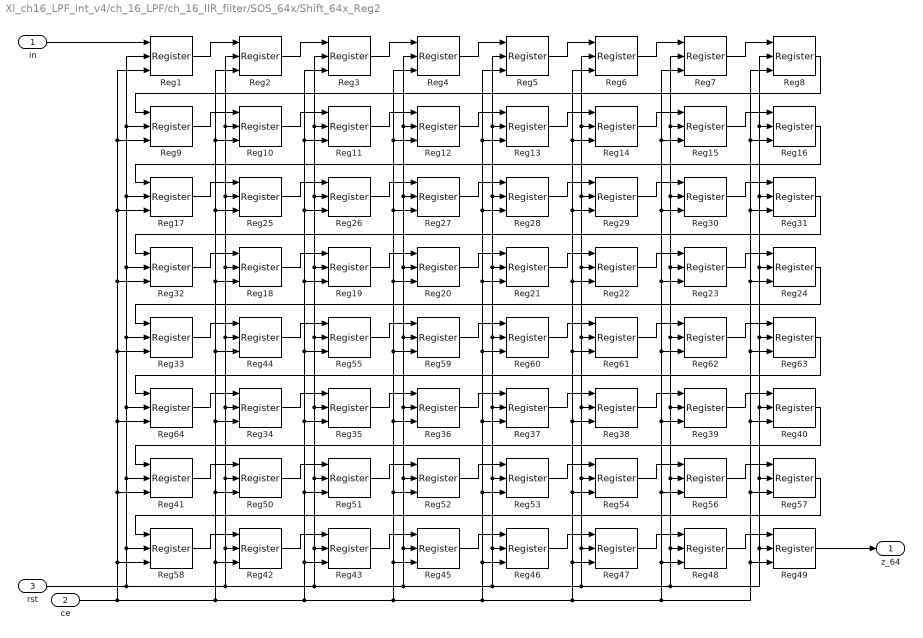
== system Xl_ch16_LPF_int_v4/ch_16_LPF/ch_16_IIR_filter/SOS_64x/Shift_64x_Reg2 ==
  in : Inport  OutDataType=fixdt(1, 16)  OutScaling=2^0
  ce : Inport  Port=2  OutDataType=fixdt(1, 16)  OutScaling=2^0
  rst : Inport  Port=3  OutDataType=fixdt(1, 16)  OutScaling=2^0
  Reg{1..64} (64 alike) : xbsIndex_r4/Register  init=0  rst=on  en=on  dbl_ovrd=off  block_type=register
      settings: block_version=12.2
  z_64 : Outport  OutDataType=fixdt(1, 16)  OutScaling=2^0
  wires:
  ce/1 -> Reg58/3, Reg41/3, Reg64/3, Reg33/3, Reg32/3, Reg17/3, Reg9/3, Reg1/3, Reg42/3, Reg50/3, Reg34/3, Reg44/3, Reg18/3, Reg25/3, Reg10/3, Reg2/3, Reg43/3, Reg51/3, Reg35/3, Reg55/3, Reg19/3, Reg26/3, Reg11/3, Reg3/3, Reg45/3, Reg52/3, Reg36/3, Reg59/3, Reg20/3, Reg27/3, Reg12/3, Reg4/3, Reg46/3, Reg53/3, Reg37/3, Reg60/3, Reg21/3, Reg28/3, Reg13/3, Reg5/3, Reg47/3, Reg54/3, Reg38/3, Reg61/3, Reg22/3, Reg29/3, Reg14/3, Reg6/3, Reg48/3, Reg56/3, Reg39/3, Reg62/3, Reg23/3, Reg30/3, Reg15/3, Reg7/3, Reg49/3, Reg57/3, Reg40/3, Reg63/3, Reg24/3, Reg31/3, Reg16/3, Reg8/3
  rst/1 -> Reg58/2, Reg41/2, Reg64/2, Reg33/2, Reg32/2, Reg17/2, Reg9/2, Reg1/2, Reg42/2, Reg50/2, Reg34/2, Reg44/2, Reg18/2, Reg25/2, Reg10/2, Reg2/2, Reg11/2, Reg3/2, Reg26/2, Reg19/2, Reg55/2, Reg35/2, Reg51/2, Reg43/2, Reg45/2, Reg52/2, Reg36/2, Reg59/2, Reg20/2, Reg27/2, Reg12/2, Reg4/2, Reg46/2, Reg53/2, Reg37/2, Reg60/2, Reg21/2, Reg28/2, Reg13/2, Reg5/2, Reg47/2, Reg54/2, Reg38/2, Reg61/2, Reg22/2, Reg29/2, Reg14/2, Reg6/2, Reg48/2, Reg56/2, Reg39/2, Reg62/2, Reg23/2, Reg30/2, Reg15/2, Reg7/2, Reg49/2, Reg57/2, Reg40/2, Reg63/2, Reg24/2, Reg31/2, Reg16/2, Reg8/2
  Reg49/1 -> z_64/1
  Reg24/1 -> Reg33/1
  Reg40/1 -> Reg41/1
  Reg57/1 -> Reg58/1
  Reg58/1 -> Reg42/1
  Reg42/1 -> Reg43/1
  Reg43/1 -> Reg45/1
  Reg45/1 -> Reg46/1
  Reg46/1 -> Reg47/1
  Reg47/1 -> Reg48/1
  Reg48/1 -> Reg49/1
  Reg41/1 -> Reg50/1
  Reg50/1 -> Reg51/1
  Reg51/1 -> Reg52/1
  Reg52/1 -> Reg53/1
  Reg53/1 -> Reg54/1
  Reg54/1 -> Reg56/1
  Reg56/1 -> Reg57/1
  Reg63/1 -> Reg64/1
  Reg64/1 -> Reg34/1
  Reg34/1 -> Reg35/1
  Reg35/1 -> Reg36/1
  Reg36/1 -> Reg37/1
  Reg37/1 -> Reg38/1
  Reg38/1 -> Reg39/1
  Reg39/1 -> Reg40/1
  Reg33/1 -> Reg44/1
  Reg44/1 -> Reg55/1
  Reg55/1 -> Reg59/1
  Reg59/1 -> Reg60/1
  Reg60/1 -> Reg61/1
  Reg61/1 -> Reg62/1
  Reg62/1 -> Reg63/1
  Reg16/1 -> Reg17/1
  Reg31/1 -> Reg32/1
  Reg32/1 -> Reg18/1
  Reg18/1 -> Reg19/1
  Reg19/1 -> Reg20/1
  Reg20/1 -> Reg21/1
  Reg21/1 -> Reg22/1
  Reg22/1 -> Reg23/1
  Reg23/1 -> Reg24/1
  Reg17/1 -> Reg25/1
  Reg25/1 -> Reg26/1
  Reg26/1 -> Reg27/1
  Reg27/1 -> Reg28/1
  Reg28/1 -> Reg29/1
  Reg29/1 -> Reg30/1
  Reg30/1 -> Reg31/1
  Reg8/1 -> Reg9/1
  Reg9/1 -> Reg10/1
  Reg10/1 -> Reg11/1
  Reg11/1 -> Reg12/1
  Reg12/1 -> Reg13/1
  Reg13/1 -> Reg14/1
  Reg14/1 -> Reg15/1
  Reg15/1 -> Reg16/1
  in/1 -> Reg1/1
  Reg1/1 -> Reg2/1
  Reg2/1 -> Reg3/1
  Reg3/1 -> Reg4/1
  Reg4/1 -> Reg5/1
  Reg5/1 -> Reg6/1
  Reg6/1 -> Reg7/1
  Reg7/1 -> Reg8/1

== system Xl_ch16_LPF_int_v4/ch_16_LPF/ch_16_IIR_filter/SOS_64x_IO_ctrl/ch_16_filt_sync ==
  note: Keep fsync phase consistent
      | with gc/a2c/a3c  phase
  cnt6b : Inport  OutDataType=fixdt(1, 16)  OutScaling=2^0
  AeqB : xbsIndex_r4/Relational  mode=a=b  en=off  latency=0  dbl_ovrd=off  block_type=relational
      settings: block_version=12.2
  Constant : xbsIndex_r4/Constant  arith_type=Unsigned  const=2  n_bits=2  bin_pt=0  explicit_period=off  period=1  equ=P=C  opselect=C  inp2=PCIN>>17  opr=+  inp1=P  carry=CIN  dbl_ovrd=off  block_type=constant
      settings: block_version=12.2
  Slice_2LSB : xbsIndex_r4/Slice  nbits=2  boolean_output=off  mode=Lower Bit Location + Width  bit1=0  base1=MSB of Input  bit0=0  base0=LSB of Input  dbl_ovrd=off  block_type=slice
      settings: block_version=12.2
  fsync : Outport  OutDataType=fixdt(1, 16)  OutScaling=2^0
  wires:
  cnt6b/1 -> Slice_2LSB/1
  Slice_2LSB/1 -> AeqB/1
  AeqB/1 -> fsync/1
  Constant/1 -> AeqB/2

== system Xl_ch16_LPF_int_v4/ch_16_LPF/ch_16_IIR_filter/SOS_64x_IO_ctrl/ch_16_filt_sync1 ==
  note: Keep fsync phase consistent
      | with gc/a2c/a3c  phase
  cnt6b : Inport  OutDataType=fixdt(1, 16)  OutScaling=2^0
  AeqB : xbsIndex_r4/Relational  mode=a=b  en=off  latency=0  dbl_ovrd=off  block_type=relational
      settings: block_version=12.2
  Constant : xbsIndex_r4/Constant  arith_type=Unsigned  const=3  n_bits=2  bin_pt=0  explicit_period=off  period=1  equ=P=C  opselect=C  inp2=PCIN>>17  opr=+  inp1=P  carry=CIN  dbl_ovrd=off  block_type=constant
      settings: block_version=12.2
  Slice_2LSB : xbsIndex_r4/Slice  nbits=2  boolean_output=off  mode=Lower Bit Location + Width  bit1=0  base1=MSB of Input  bit0=0  base0=LSB of Input  dbl_ovrd=off  block_type=slice
      settings: block_version=12.2
  fsync : Outport  OutDataType=fixdt(1, 16)  OutScaling=2^0
  wires:
  cnt6b/1 -> Slice_2LSB/1
  Slice_2LSB/1 -> AeqB/1
  AeqB/1 -> fsync/1
  Constant/1 -> AeqB/2

== system Xl_ch16_LPF_int_v4/ch_16_LPF/ch_16_IIR_filter/Demux_16x/dec_4bit/bus2bit ==
  d : Inport
  extraxt_b0 : xbsIndex_r4/Slice  nbits=1  boolean_output=on  mode=Lower Bit Location + Width  bit1=0  base1=MSB of Input  bit0=0  base0=LSB of Input  dbl_ovrd=off  block_type=slice
      settings: block_version=12.2
  extraxt_b1 : xbsIndex_r4/Slice  nbits=1  boolean_output=on  mode=Lower Bit Location + Width  bit1=0  base1=MSB of Input  bit0=1  base0=LSB of Input  dbl_ovrd=off  block_type=slice
      settings: block_version=12.2
  extraxt_b2 : xbsIndex_r4/Slice  nbits=1  boolean_output=on  mode=Lower Bit Location + Width  bit1=0  base1=MSB of Input  bit0=2  base0=LSB of Input  dbl_ovrd=off  block_type=slice
      settings: block_version=12.2
  extraxt_b3 : xbsIndex_r4/Slice  nbits=1  boolean_output=on  mode=Lower Bit Location + Width  bit1=0  base1=MSB of Input  bit0=3  base0=LSB of Input  dbl_ovrd=off  block_type=slice
      settings: block_version=12.2
  b0 : Outport
  b1 : Outport  Port=2
  b2 : Outport  Port=3
  b3 : Outport  Port=4
  wires:
  d/1 -> extraxt_b0/1, extraxt_b1/1, extraxt_b3/1, extraxt_b2/1
  extraxt_b0/1 -> b0/1
  extraxt_b1/1 -> b1/1
  extraxt_b2/1 -> b2/1
  extraxt_b3/1 -> b3/1

== system Xl_ch16_LPF_int_v4/ch_16_LPF/ch_16_IIR_filter/Demux_16x/dec_4bit/neg_bus2bit ==
  d : Inport
  extraxt_b0 : xbsIndex_r4/Slice  nbits=1  boolean_output=on  mode=Lower Bit Location + Width  bit1=0  base1=MSB of Input  bit0=0  base0=LSB of Input  dbl_ovrd=off  block_type=slice
      settings: block_version=12.2
  extraxt_b1 : xbsIndex_r4/Slice  nbits=1  boolean_output=on  mode=Lower Bit Location + Width  bit1=0  base1=MSB of Input  bit0=1  base0=LSB of Input  dbl_ovrd=off  block_type=slice
      settings: block_version=12.2
  extraxt_b2 : xbsIndex_r4/Slice  nbits=1  boolean_output=on  mode=Lower Bit Location + Width  bit1=0  base1=MSB of Input  bit0=2  base0=LSB of Input  dbl_ovrd=off  block_type=slice
      settings: block_version=12.2
  extraxt_b3 : xbsIndex_r4/Slice  nbits=1  boolean_output=on  mode=Lower Bit Location + Width  bit1=0  base1=MSB of Input  bit0=3  base0=LSB of Input  dbl_ovrd=off  block_type=slice
      settings: block_version=12.2
  b0 : Outport
  b1 : Outport  Port=2
  b2 : Outport  Port=3
  b3 : Outport  Port=4
  wires:
  extraxt_b3/1 -> b3/1
  extraxt_b2/1 -> b2/1
  extraxt_b1/1 -> b1/1
  extraxt_b0/1 -> b0/1
  d/1 -> extraxt_b2/1, extraxt_b3/1, extraxt_b1/1, extraxt_b0/1
